simulink library "SkywardBLIMP"  (R2014a)
settings: Solver=ode45  StartTime=0.0  StopTime=10.0  RelTol=1e-3
settings Model: Creator=Francescodario  LastModifiedBy=Francescodario

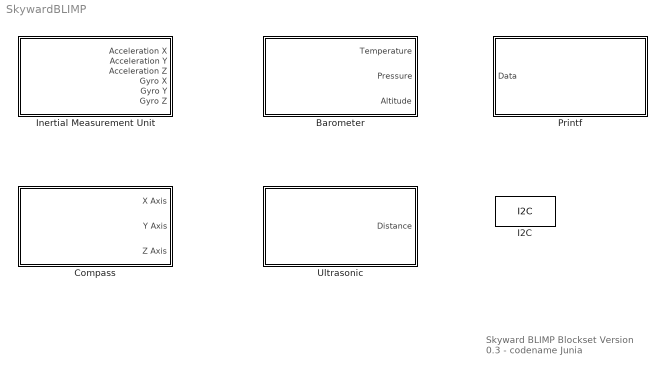
== system SkywardBLIMP ==
  note: Skyward BLIMP Blockset
      | Version 0.3 - codename Junia
  Barometer : Subsystem  mask(Barometer){}
      mask help:
      | This block drive the Bosch BMP085 barometer connected trought I2C to an Arduino Board.
      | Temperature is given in centigrade degrees, pressure in millibar and altitude in meters.
  Compass : Subsystem  mask(Compass){}
      mask help:
      | This block will drive the HMC5883L magnetometer connected to an Arduino
      | board trought I2C.
      | It will give back the normalized magnetic field on the three axis becuase
      | Aureliano Rivolta wants it this way.
      | Thanks to Silvano "Redman" Seva for helping me in the implementation of
      | this block.
  I2C : S-Function  FunctionName=I2C  SFunctionModules='I2C_wrapper'  EnableBusSupport=off  mask(I2C){}
      mask help: This block simply include the Wire library to the model.
  Inertial Measurement Unit : Subsystem  mask(Inertial Measuremente Unit){}
      mask help:
      | This block will drive the MPU6050 IMU connected to an Arduino Board.
      | The Acceleration is given back in "g", the angular velocity in degrees per second (deg/s)
  Printf : Subsystem  mask(printf){}
      mask help:
      | This block simply send data to Arduino serial port as formatted text.
      | Useful for reading sensors.
  Ultrasonic : Subsystem  mask(Ultrasonic){}
      mask help:
      | This block will drive the HCSR-04 ultrasonic sensor.
      | Distance is given back in centimeters.
      | TrigPin = 3 (Digital)
      | EchoPin = 2 (Digital)

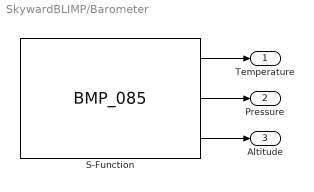
== system SkywardBLIMP/Barometer ==
  S-Function : S-Function  FunctionName=BMP_085  SFunctionModules='BMP_085_wrapper'  EnableBusSupport=off
  Temperature : Outport
  Pressure : Outport  Port=2
  Altitude : Outport  Port=3
  wires:
  S-Function/2 -> Pressure/1
  S-Function/3 -> Altitude/1
  S-Function/1 -> Temperature/1

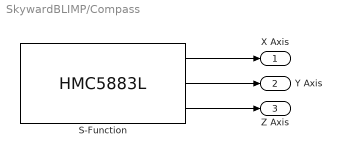
== system SkywardBLIMP/Compass ==
  S-Function : S-Function  FunctionName=HMC5883L  SFunctionModules='HMC5883L_wrapper'  EnableBusSupport=off
  X Axis : Outport
  Y Axis : Outport  Port=2
  Z Axis : Outport  Port=3
  wires:
  S-Function/3 -> Z Axis/1
  S-Function/2 -> Y Axis/1
  S-Function/1 -> X Axis/1

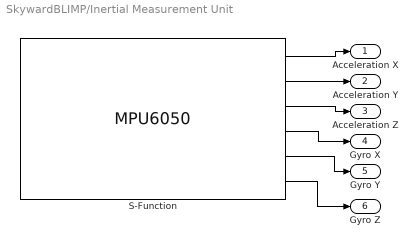
== system SkywardBLIMP/Inertial Measurement Unit ==
  S-Function : S-Function  FunctionName=MPU6050  SFunctionModules='MPU6050_wrapper'  EnableBusSupport=off
  Acceleration X : Outport
  Acceleration Y : Outport  Port=2
  Acceleration Z : Outport  Port=3
  Gyro X : Outport  Port=4
  Gyro Y : Outport  Port=5
  Gyro Z : Outport  Port=6
  wires:
  S-Function/6 -> Gyro Z/1
  S-Function/5 -> Gyro Y/1
  S-Function/2 -> Acceleration Y/1
  S-Function/1 -> Acceleration X/1
  S-Function/4 -> Gyro X/1
  S-Function/3 -> Acceleration Z/1

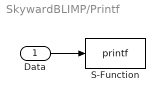
== system SkywardBLIMP/Printf ==
  Data : Inport
  S-Function : S-Function  FunctionName=printf  SFunctionModules='printf_wrapper'  EnableBusSupport=off
  wires:
  Data/1 -> S-Function/1

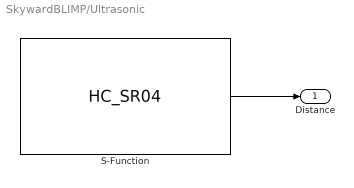
== system SkywardBLIMP/Ultrasonic ==
  S-Function : S-Function  FunctionName=HC_SR04  SFunctionModules='HC_SR04_wrapper'  EnableBusSupport=off
  Distance : Outport
  wires:
  S-Function/1 -> Distance/1
